simulink model "MALE_UAV_ENGINE"  (R2026a)
settings: Solver=ode45  StopTime=60
(part 2 of 2)

== matlab function MALE_UAV_ENGINE/Fault_Detection/Fault_Classifier ==
  data: CHT_R input double size=1; Fault_Code output double size=1; EGT_R input double size=1; OilP_R input double size=1; OilT_R input double size=1; Fuel_R input double size=1; CHT_Z input double size=1; EGT_Z input double size=1; OilP_Z input double size=1; OilT_Z input double size=1; Fuel_Z input double size=1; Vibration input double size=1; RPM input double size=1; Engine_Load input double size=1; Injection_Timing input double size=1; Battery_Voltage input double size=1; Alternator_Current input double size=1; Fault_Severity output double size=1; Fault_Confidence output double size=1; Fault_Evidence output double size=1
function [Fault_Code, Fault_Severity, Fault_Confidence, Fault_Evidence] = fcn(CHT_R, EGT_R, OilP_R, OilT_R, Fuel_R, CHT_Z, EGT_Z, OilP_Z, OilT_Z, Fuel_Z, Vibration, RPM, Engine_Load, Injection_Timing, Battery_Voltage, Alternator_Current)
best = 0;
code = 0;

aCHT = abs(CHT_Z);
aEGT = abs(EGT_Z);
aOilP = abs(OilP_Z);
aOilT = abs(OilT_Z);
aFuel = abs(Fuel_Z);

lowOilP = max(-OilP_Z,0);
highOilT = max(OilT_Z,0);
highCHT = max(CHT_Z,0);
highEGT = max(EGT_Z,0);

% Existing baseline scores
score1 = 0.40*min(aFuel,2)/2 + 0.35*min(aEGT,3)/3 + 0.25*min(max(Vibration-1.2,0),2)/2;
if aFuel < 0.5
    if aEGT < 0.5
        score1 = 0;
    end
end

score2 = 0.75*min(aFuel,2)/2 + 0.20*min(aEGT,4)/4 + 0.05*min(abs(Engine_Load-0.5),0.5)/0.5;

timing_error = abs(Injection_Timing-20);
score3 = 0.80*min(timing_error,8)/8 + 0.20*min(aEGT,4)/4;

score4 = 0.65*min(lowOilP,2)/2 + 0.35*min(highOilT,2)/2;

score5 = 0;
sensor_count = 0;
if aCHT > 2
    sensor_count = sensor_count + 1;
end
if aEGT > 2
    sensor_count = sensor_count + 1;
end
if aOilP > 2
    sensor_count = sensor_count + 1;
end
if aOilT > 2
    sensor_count = sensor_count + 1;
end
if aFuel > 2
    sensor_count = sensor_count + 1;
end
if sensor_count >= 3
    score5 = 0.45 + 0.15*(sensor_count-3);
    score5 = min(score5,1);
elseif sensor_count == 2
    score5 = 0.20;
end

score6 = 0.50*min(aEGT,3)/3 + 0.35*min(max(Vibration-1.2,0),2)/2 + 0.15*min(aFuel,4)/4;
if aFuel >= 1.5
    score6 = score6*0.50;
end

score7 = 0.50*min(highCHT,3)/3 + 0.35*min(highEGT,3)/3 + 0.15*min(highOilT,3)/3;

thermal_count = 0;
if highCHT > 1
    thermal_count = thermal_count + 1;
end
if highEGT > 1
    thermal_count = thermal_count + 1;
end
if highOilT > 1
    thermal_count = thermal_count + 1;
end
if thermal_count < 2
    score7 = score7*0.30;
end

score8 = min(max(Vibration-1.2,0),3)/3;
if aEGT > 1
    score8 = score8*0.25;
elseif aFuel > 1
    score8 = score8*0.25;
elseif highCHT > 1
    score8 = score8*0.25;
end

% Signature-aware selection
override = 0;
overrideScore = 0;

% Fault 5: sensor fault - contradictory CHT/EGT/OilP signs
if CHT_Z > 2
    if EGT_Z < -1
        if OilP_Z < -3
            override = 5;
            overrideScore = 0.90;
        end
    end
end

% Fault 7: overheating - CHT and EGT both strongly positive
if override == 0
    if CHT_Z > 3
        if EGT_Z > 2
            override = 7;
            overrideScore = 0.90;
        end
    end
end

% Fault 1 / 6 separation using measured signatures
if override == 0
    if EGT_Z > 2.97
        if Fuel_Z < -0.10
            if Vibration > 2.60
                override = 1;
                overrideScore = 0.90;
            end
        end
    end
end

% Combustion instability
if override == 0
    if EGT_Z > 2
        if Fuel_Z < -0.10
            override = 6;
            overrideScore = 0.90;
        end
    end
end

% Fault 2: injector - EGT positive with fuel increase
if override == 0
    if EGT_Z > 1
        if Fuel_Z > 0.30
            override = 2;
            overrideScore = 0.90;
        end
    end
end

if override ~= 0
    code = override;
    best = overrideScore;
else
    if score1 > best
        best = score1;
        code = 1;
    end
    if score2 > best
        best = score2;
        code = 2;
    end
    if score3 > best
        best = score3;
        code = 3;
    end
    if score4 > best
        best = score4;
        code = 4;
    end
    if score5 > best
        best = score5;
        code = 5;
    end
    if score6 > best
        best = score6;
        code = 6;
    end
    if score7 > best
        best = score7;
        code = 7;
    end
    if score8 > best
        best = score8;
        code = 8;
    end
end

Fault_Code = code;
Fault_Evidence = best;

if best < 0.35
    Fault_Code = 0;
    Fault_Severity = 0;
    Fault_Confidence = 0;
else
    Fault_Severity = best;
    Fault_Confidence = best;
end
end

== matlab function MALE_UAV_ENGINE/Degradation_Model/Degradation_Rate_Model ==
  data: Fault_Severity input; Thermal_Rate output; Fault_Code input; CHT_Z input; EGT_Z input; OilP_Z input; OilT_Z input; Fuel_Z input; Vibration input; RPM input; Engine_Load input; Lubrication_Rate output; Combustion_Rate output; Mechanical_Rate output; Electrical_Rate output; Overall_Rate output
function [Thermal_Rate, Lubrication_Rate, Combustion_Rate, Mechanical_Rate, Electrical_Rate, Overall_Rate] = ...
fcn(Fault_Severity, Fault_Code, CHT_Z, EGT_Z, OilP_Z, OilT_Z, Fuel_Z, Vibration, RPM, Engine_Load)
% SIH26 Digital Twin
% Degradation Model V1
% Converts abnormal operating evidence into
% accumulated degradation rates.
%
% V1 = engineering/heuristic model.
% Calibration and validation are required.

    Fault_Severity = max(0, min(1, Fault_Severity));
    Fault_Code = max(0, round(Fault_Code));
    RPM = max(0, RPM);
    Engine_Load = max(0, min(1, Engine_Load));

    %% Normalized abnormality evidence
    c = min(abs(CHT_Z) / 3, 1);
    e = min(abs(EGT_Z) / 3, 1);
    op = min(abs(OilP_Z) / 3, 1);
    ot = min(abs(OilT_Z) / 3, 1);
    f = min(abs(Fuel_Z) / 3, 1);

    %% Vibration abnormality
    vibration_abnormal = min(max(Vibration - 1.2, 0) / 3, 1);

    %% Operating stress
    rpm_factor = min(RPM / 5800, 1);
    load_factor = Engine_Load;
    operating_stress = 0.5 * rpm_factor + 0.5 * load_factor;

    %% Thermal degradation
    Thermal_Rate = ...
        2e-6 * (0.45*c + 0.40*e + 0.15*ot) ...
        * (0.5 + 0.5*operating_stress);

    %% Lubrication degradation
    Lubrication_Rate = ...
        2e-6 * (0.70*op + 0.30*ot) ...
        * (0.5 + 0.5*load_factor);

    %% Combustion degradation
    Combustion_Rate = ...
        2e-6 * (0.45*e + 0.35*f + 0.20*Fault_Severity) ...
        * (0.5 + 0.5*load_factor);

    %% Mechanical degradation
    Mechanical_Rate = ...
        2e-6 * (0.55*vibration_abnormal + 0.25*e + 0.20*Fault_Severity) ...
        * (0.5 + 0.5*rpm_factor);

    %% Electrical degradation
    Electrical_Rate = 0.5e-6 * Fault_Severity;

    %% Fault-specific acceleration
    switch Fault_Code
        case 1
            Combustion_Rate = Combustion_Rate * 1.50;
        case 2
            Combustion_Rate = Combustion_Rate * 1.40;
        case 3
            Combustion_Rate = Combustion_Rate * 1.30;
        case 4
            Lubrication_Rate = Lubrication_Rate * 1.60;
        case 5
            Electrical_Rate = Electrical_Rate * 1.20;
        case 6
            Combustion_Rate = Combustion_Rate * 1.50;
        case 7
            Thermal_Rate = Thermal_Rate * 1.70;
        case 8
            Mechanical_Rate = Mechanical_Rate * 1.70;
    end

    %% Overall degradation rate
    Overall_Rate = ...
        0.25*Thermal_Rate + ...
        0.20*Lubrication_Rate + ...
        0.25*Combustion_Rate + ...
        0.20*Mechanical_Rate + ...
        0.10*Electrical_Rate;

    Thermal_Rate = max(0, Thermal_Rate);
    Lubrication_Rate = max(0, Lubrication_Rate);
    Combustion_Rate = max(0, Combustion_Rate);
    Mechanical_Rate = max(0, Mechanical_Rate);
    Electrical_Rate = max(0, Electrical_Rate);
    Overall_Rate = max(0, Overall_Rate);

end

== matlab function MALE_UAV_ENGINE/RUL_Model/RUL_Estimator ==
  data: Degradation input; RUL_Normalized output; Degradation_Rate input; Health_Index input; Fault_Severity input; Engine_Load input; RPM input; RUL_Hours output; RUL_Confidence output; Life_State output
function [RUL_Normalized, RUL_Hours, RUL_Confidence, Life_State] = ...
fcn(Degradation, Degradation_Rate, Health_Index, Fault_Severity, Engine_Load, RPM)
% SIH26 Digital Twin
% RUL Estimator V1
%
% V1 uses degradation-rate extrapolation.
% This is an architectural prototype and must be
% calibrated against real degradation/failure datasets
% before operational use.

    %% Input protection
    Degradation = max(0, min(1, Degradation));
    Degradation_Rate = max(0, Degradation_Rate);
    Health_Index = max(0, min(1, Health_Index));
    Fault_Severity = max(0, min(1, Fault_Severity));
    Engine_Load = max(0, min(1, Engine_Load));
    RPM = max(0, RPM);

    %% Remaining degradation margin
    degradation_limit = 1.0;
    remaining_margin = max(0, degradation_limit - Degradation);

    %% Minimum rate floor prevents infinite RUL
    rate_floor = 1e-8;
    effective_rate = max(Degradation_Rate, rate_floor);

    %% Base RUL in model time units
    RUL_time_units = remaining_margin / effective_rate;

    %% Convert model time to hours.
    % V1 assumes simulation time is seconds.
    RUL_Hours = RUL_time_units / 3600;

    %% Operational severity adjustment
    stress_factor = 1 + 0.5*Engine_Load + 0.3*(RPM/5800);
    stress_factor = max(1, stress_factor);

    RUL_Hours = RUL_Hours / stress_factor;

    %% Fault severity penalty
    RUL_Hours = RUL_Hours * (1 - 0.30*Fault_Severity);

    %% Bound RUL
    RUL_Hours = max(0, RUL_Hours);

    %% Normalized RUL
    reference_life_hours = 1000;
    RUL_Normalized = RUL_Hours / reference_life_hours;
    RUL_Normalized = max(0, min(1, RUL_Normalized));

    %% Confidence estimate
    % Confidence is deliberately conservative when
    % degradation evidence is weak or rate is tiny.
    rate_strength = min(1, Degradation_Rate / 1e-5);
    evidence_strength = max(Fault_Severity, 1-Health_Index);

    RUL_Confidence = ...
        0.60*rate_strength + ...
        0.40*evidence_strength;

    RUL_Confidence = max(0, min(1, RUL_Confidence));

    %% Life state
    if Degradation < 0.20
        Life_State = 1;
    elseif Degradation < 0.50
        Life_State = 2;
    elseif Degradation < 0.75
        Life_State = 3;
    else
        Life_State = 4;
    end

    %%
    % Life_State:
    % 1 = Healthy
    % 2 = Degrading
    % 3 = Critical
    % 4 = End-of-life boundary
    %
end

== matlab function MALE_UAV_ENGINE/Fault_Injection/Fault_Injection_Model ==
  data: RPM_i input; RPM_o output; CHT_i input; EGT_i input; OilP_i input; OilT_i input; FuelFlow_i input; BatteryVoltage_i input; AlternatorCurrent_i input; InjectionTiming_i input; Vibration_i input; Enable input; Fault_Type input; Severity input; CHT_o output; EGT_o output; OilP_o output; OilT_o output; FuelFlow_o output; BatteryVoltage_o output; AlternatorCurrent_o output; InjectionTiming_o output; Vibration_o output
function [RPM_o, CHT_o, EGT_o, OilP_o, OilT_o, FuelFlow_o, BatteryVoltage_o, AlternatorCurrent_o, InjectionTiming_o, Vibration_o] = fcn(RPM_i, CHT_i, EGT_i, OilP_i, OilT_i, FuelFlow_i, BatteryVoltage_i, AlternatorCurrent_i, InjectionTiming_i, Vibration_i, Enable, Fault_Type, Severity)

% SIH26 Digital Twin - Fault Injection Layer V1

Severity = max(0, min(1, Severity));
Enable = Enable > 0.5;

% Default pass-through
RPM_o = RPM_i;
CHT_o = CHT_i;
EGT_o = EGT_i;
OilP_o = OilP_i;
OilT_o = OilT_i;
FuelFlow_o = FuelFlow_i;
BatteryVoltage_o = BatteryVoltage_i;
AlternatorCurrent_o = AlternatorCurrent_i;
InjectionTiming_o = InjectionTiming_i;
Vibration_o = Vibration_i;

if Enable
    switch round(Fault_Type)
        case 1
            % Misfire
            EGT_o = EGT_i * (1 + 0.15 * Severity);
            FuelFlow_o = FuelFlow_i * (1 - 0.10 * Severity);
            Vibration_o = Vibration_i + 1.5 * Severity;

        case 2
            % Injector abnormality
            FuelFlow_o = FuelFlow_i * (1 + 0.25 * Severity);
            EGT_o = EGT_i * (1 + 0.10 * Severity);

        case 3
            % Coding degradation / injection timing deviation
            InjectionTiming_o = InjectionTiming_i + 10 * Severity;
            EGT_o = EGT_i * (1 + 0.08 * Severity);

        case 4
            % Lubrication issue
            OilP_o = OilP_i * (1 - 0.60 * Severity);
            OilT_o = OilT_i + 40 * Severity;

        case 5
            % Sensor fault
            CHT_o = CHT_i + 50 * Severity;
            EGT_o = EGT_i - 80 * Severity;
            OilP_o = OilP_i * (1 - 0.30 * Severity);

        case 6
            % Combustion instability
            EGT_o = EGT_i * (1 + 0.12 * Severity);
            FuelFlow_o = FuelFlow_i * (1 - 0.08 * Severity);
            Vibration_o = Vibration_i + 1.0 * Severity;

        case 7
            % Overheating
            CHT_o = CHT_i + 80 * Severity;
            EGT_o = EGT_i + 150 * Severity;
            OilT_o = OilT_i + 50 * Severity;

        case 8
            % Abnormal vibration
            Vibration_o = Vibration_i + 4.0 * Severity;
    end
end

end

== matlab function MALE_UAV_ENGINE/Engine_Core/Fuel_System/MATLAB Function ==
  data: Air_Mass_Flow input; Fuel_Flow output; Engine_Load input; Injection_Timing input
function Fuel_Flow = fcn(Air_Mass_Flow, Engine_Load, Injection_Timing)

% SIH26 Digital Twin
% Fuel System Model V1

    %% Model parameters
    target_AFR = 14.7;
    combustion_efficiency = 0.98;

    %% Input protection
    Air_Mass_Flow = max(0, Air_Mass_Flow);
    Engine_Load = max(0, min(1, Engine_Load));

    %% Injection timing effect
    optimal_timing = 20;
    timing_sensitivity = 0.001;

    timing_error = Injection_Timing - optimal_timing;

    timing_efficiency = ...
        max(0, 1 - timing_sensitivity * timing_error^2);

    %% Fuel flow
    Fuel_Flow = ...
        (Air_Mass_Flow / target_AFR) ...
        * combustion_efficiency ...
        * timing_efficiency ...
        * Engine_Load;

end

== matlab function MALE_UAV_ENGINE/Engine_Core/Air_Charge/MATLAB Function ==
  data: Throttle input; MAP output; RPM input; Ambient_Pressure input; Ambient_Temperature input; Air_Mass_Flow output
function [MAP, Air_Mass_Flow] = fcn(Throttle, RPM, Ambient_Pressure, Ambient_Temperature)

% SIH26 Digital Twin
% Air-Charge Model V1

    %% Constants
    R_air = 287.05;                 % J/(kg*K)
    volumetric_efficiency = 0.80;   % V1 assumption
    displacement = 1.352e-3;        % m^3

    %% Input protection
    Throttle = max(0, min(1, Throttle));
    RPM = max(0, RPM);

    %% Manifold Absolute Pressure
    MAP = Ambient_Pressure * Throttle;

    %% Air mass flow
    Air_Mass_Flow = ...
        (MAP * displacement / ...
        (R_air * Ambient_Temperature)) ...
        * (RPM / 120) ...
        * volumetric_efficiency;

end

== matlab function MALE_UAV_ENGINE/Engine_Core/Combustion/Combustion_Model ==
  data: Fuel_Flow input; Indicated_Power output; Injection_Timing input
function Indicated_Power = fcn(Fuel_Flow, Injection_Timing)

% SIH26 Digital Twin
% Combustion Model
%
% V1 implementation:
%   Fuel energy -> indicated power
%   Injection timing modifies combustion effectiveness.
%
% Architecture:
%   Keep this interface stable while the internal
%   combustion model is upgraded from V1 -> V5.

    %% V1 model parameters

    lower_heating_value = 43e6;     % J/kg
    indicated_efficiency = 0.30;

    optimal_timing = 20;             % deg
    timing_sensitivity = 0.001;

    %% Input protection

    Fuel_Flow = max(0, Fuel_Flow);

    %% Injection timing effect

    timing_error = ...
        Injection_Timing - optimal_timing;

    timing_efficiency = ...
        max(0, ...
        1 - timing_sensitivity * timing_error^2);

    %% Chemical energy rate

    fuel_energy_rate = ...
        Fuel_Flow * lower_heating_value;

    %% Indicated power

    Indicated_Power = ...
        fuel_energy_rate ...
        * indicated_efficiency ...
        * timing_efficiency;

end

== matlab function MALE_UAV_ENGINE/Engine_Core/Torque_Power/Torque_Power_Model ==
  data: Indicated_Power input; Brake_Power output; RPM input; Torque output
function [Brake_Power, Torque] = fcn(Indicated_Power, RPM)
% SIH26 Digital Twin
% Torque and Power Model
%
% V1 implementation:
% Converts indicated power to brake power
% and calculates shaft torque.
%
% Interface is intentionally stable for V1 -> V5.

    %% V1 model parameter
    mechanical_efficiency = 0.85;

    %% Input protection
    Indicated_Power = max(0, Indicated_Power);
    RPM = max(0, RPM);

    %% Brake power
    Brake_Power = ...
        Indicated_Power * mechanical_efficiency;

    %% Angular velocity
    omega = 2 * pi * max(RPM, 1) / 60;

    %% Shaft torque
    Torque = Brake_Power / omega;

end

== matlab function MALE_UAV_ENGINE/Thermal_System/Thermal_Dynamics ==
  data: Fuel_Flow input; dCHT output; RPM input; Ambient_Temperature input; Engine_Load input; CHT input; EGT input; Oil_Temp input; dEGT output; dOil output
function [dCHT, dEGT, dOil] = fcn(Fuel_Flow, RPM, Ambient_Temperature, Engine_Load, CHT, EGT, Oil_Temp)
% SIH26 Digital Twin
% Lumped thermal dynamics model V1
%
% Outputs are temperature derivatives in K/s.
% V1 parameters are representative assumptions and
% will be calibrated against validated engine data.

    %% Physical constants
    LHV = 43e6;

    %% Input protection
    Fuel_Flow = max(0, Fuel_Flow);
    RPM = max(0, RPM);
    Engine_Load = max(0, min(1, Engine_Load));

    %% Fuel energy rate
    Fuel_Power = Fuel_Flow * LHV;

    %% Lumped thermal parameters
    CHT_capacity = 20000;
    EGT_capacity = 5000;
    Oil_capacity = 15000;

    %% Heat generation
    Q_combustion = Fuel_Power;

    Q_CHT_in = 0.08 * Q_combustion;
    Q_EGT_in = 0.30 * Q_combustion;
    Q_Oil_in = 0.04 * Q_combustion;

    %% Cooling coefficients
    CHT_cooling = (20 + 0.015 * RPM) * max(CHT - Ambient_Temperature, 0);
    Oil_cooling = (12 + 0.008 * RPM) * max(Oil_Temp - Ambient_Temperature, 0);

    %% EGT heat rejection
    EGT_cooling = (8 + 0.004 * RPM) * max(EGT - Ambient_Temperature, 0);

    %% Temperature dynamics
    dCHT = (Q_CHT_in - CHT_cooling) / CHT_capacity;
    dEGT = (Q_EGT_in - EGT_cooling) / EGT_capacity;
    dOil = (Q_Oil_in - Oil_cooling) / Oil_capacity;

end

== matlab function MALE_UAV_ENGINE/Lubrication_System/Lubrication_Model ==
  data: RPM input; Target_Pressure output; Engine_Load input; Oil_Temperature input; Oil_Flow output
function [Target_Pressure, Oil_Flow] = fcn(RPM, Engine_Load, Oil_Temperature)
% SIH26 Digital Twin
% Lubrication System V1
%
% Representative lumped lubrication model.
% Oil pressure depends on pump speed, load,
% and temperature-dependent viscosity.

    %% Input protection
    RPM = max(0, RPM);
    Engine_Load = max(0, min(1, Engine_Load));
    Oil_Temperature = max(250, Oil_Temperature);

    %% Representative oil properties
    reference_temperature = 373.15;
    reference_viscosity = 0.020;

    %% Temperature-dependent viscosity
    viscosity = reference_viscosity * exp( ...
        -0.025 * (Oil_Temperature - reference_temperature));

    viscosity = max(viscosity, 0.002);

    %% Pump behaviour
    pump_factor = RPM / 5800;
    load_factor = 0.30 + 0.70 * Engine_Load;

    %% Pressure capability
    base_pressure = 500000;
    pressure_gain = 2500000 * pump_factor * load_factor;

    viscosity_factor = reference_viscosity / viscosity;

    Target_Pressure = ...
        base_pressure + pressure_gain * viscosity_factor;

    %% Oil flow
    Oil_Flow = ...
        (0.00002 * RPM / 1000) * load_factor * viscosity_factor;

    %% Physical limits
    Target_Pressure = max(0, Target_Pressure);
    Oil_Flow = max(0, Oil_Flow);

end

== matlab function MALE_UAV_ENGINE/Electrical_System/Electrical_Model ==
  data: RPM input; Battery_Voltage output; Engine_Load input; Battery_State input; Alternator_Current output
function [Battery_Voltage, Alternator_Current] = fcn(RPM, Engine_Load, Battery_State)
% SIH26 Digital Twin
% Electrical System V1
%
% Representative electrical behaviour model.
% Intended interface remains stable for future ECU/BMS data.

    %% Input protection
    RPM = max(0, RPM);
    Engine_Load = max(0, min(1, Engine_Load));
    Battery_State = max(0, min(1, Battery_State));

    %% Battery model
    nominal_voltage = 14.0;
    internal_drop = 1.2 * (1 - Battery_State);

    %% Alternator generation
    alternator_capacity = 40;
    rpm_factor = min(RPM / 3000, 1);

    Alternator_Current = ...
        alternator_capacity * rpm_factor ...
        * (0.25 + 0.75 * Battery_State);

    %% Electrical load
    base_load = 5;
    engine_load_current = 8 * Engine_Load;

    electrical_load = base_load + engine_load_current;

    %% Battery voltage response
    charging_effect = 0.015 * Alternator_Current;
    load_effect = 0.03 * electrical_load;

    Battery_Voltage = ...
        nominal_voltage ...
        + charging_effect ...
        - load_effect ...
        - internal_drop;

    %% Physical bounds
    Battery_Voltage = max(9, min(15, Battery_Voltage));
    Alternator_Current = max(0, Alternator_Current);

end
